simulink model "openloop_simulator"  (R2017a)
settings: Solver=ode4  StartTime=0.0  StopTime=inf  FixedStep=0.1  RelTol=1e-3
libraries: realtime_pacer_lib x1
settings Model: SnapshotBufferSize=1000  SnapshotInterval=1000  Creator=Roshan  LastModifiedBy=rosha
settings RTWCC: SystemTargetFile=sldrt.tlc  TemplateMakefile=sldrt.tmf  Description=Simulink Desktop Real-Time  RTWCompilerOptimization=on
settings CodeAppCC: MaxIdLength=95
settings SimulinkDesktopRealTimeCC: TargetPreCompLibLocation=C:\Program Files\MATLAB\R2017a\toolbox\sldrt\lib\win64  SupportVariableSizeSignals=off

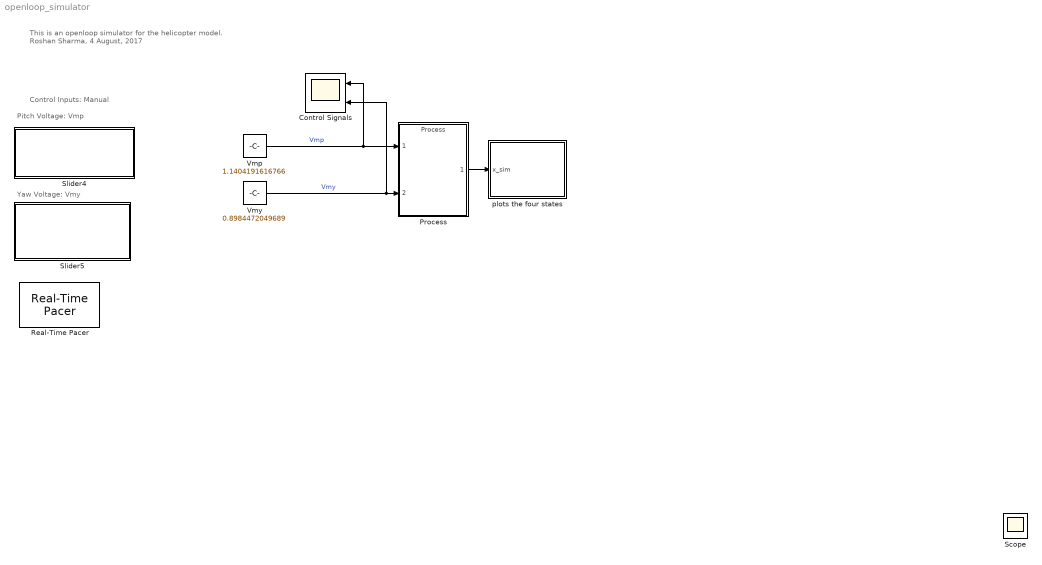
== system openloop_simulator ==
  note: Control Inputs: Manual
  note: This is an openloop simulator
      | for the helicopter model.
      | Roshan Sharma, 4 August, 2017
  note: Pitch Voltage: Vmp
  note: Yaw Voltage: Vmy
  Control Signals : Scope  NumInputPorts=2
  Process : ModelReference  ModelNameDialog=Process  ModelReferenceVersion=1.989  CopyOfModelProtected=on
  Real-Time Pacer : realtime_pacer_lib/Real-Time Pacer  simTimePerRealTime=1
  Slider4 : Subsystem  DialogController=hmiCreateDDGDialog  IsWebBlock=on  mask(MWDashboardBlock){webBlockId=d7fa2b72-57f0-4581-a642-3c1b7216c1b6, webBlockType=slider, ShowInLibBrowser=on, ShowInitialText=on, HMISrcModelName=protected_simulator}
      mask prompts: webBlockId "WebBlock Id"; webBlockType "WebBlock Type"; HMISrcModelName "Source Model"
      mask help: SimulinkHMI:dialogs:SliderDialogDesc
      mask Help: helpview([docroot '/mapfiles/simulink.map'], 'hmi_slider')
      mask Display:
      | if strcmp(get_param(bdroot(gcb),'BlockDiagramType'), 'library')
      |     image([(matlabroot) '/toolbox/simulink/hmi/icons/Slider.png']);
      | end
  Slider5 : Subsystem  DialogController=hmiCreateDDGDialog  IsWebBlock=on  mask(MWDashboardBlock){webBlockId=2da1ea5c-a5f5-4938-b925-ee22b86d0a23, webBlockType=slider, ShowInLibBrowser=on, ShowInitialText=on, HMISrcModelName=protected_simulator}
      mask prompts: webBlockId "WebBlock Id"; webBlockType "WebBlock Type"; HMISrcModelName "Source Model"
      mask help: SimulinkHMI:dialogs:SliderDialogDesc
      mask Help: helpview([docroot '/mapfiles/simulink.map'], 'hmi_slider')
      mask Display:
      | if strcmp(get_param(bdroot(gcb),'BlockDiagramType'), 'library')
      |     image([(matlabroot) '/toolbox/simulink/hmi/icons/Slider.png']);
      | end
  Vmp : Constant  Value=1.1404191616766
  Vmy : Constant  Value=0.8984472049689
  plots the four states : Subsystem
  Scope : Scope
  wires:
  Vmp/1 -> Process/1, Control Signals/1  "Vmp"
  Vmy/1 -> Process/2, Control Signals/2  "Vmy"
  Process/1 -> plots the four states/1(x_sim)

== system openloop_simulator/Slider4 ==

== system openloop_simulator/Slider5 ==

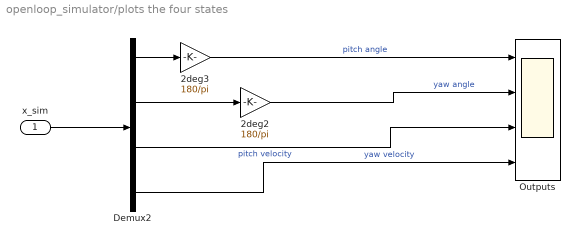
== system openloop_simulator/plots the four states ==
  x_sim : Inport
  2deg2 : Gain  Gain=180/pi
  2deg3 : Gain  Gain=180/pi
  Demux2 : Demux
  Outputs : Scope  NumInputPorts=4
  wires:
  x_sim/1 -> Demux2/1
  Demux2/1 -> 2deg3/1
  Demux2/2 -> 2deg2/1
  2deg3/1 -> Outputs/1  "pitch angle"
  2deg2/1 -> Outputs/2  "yaw angle"
  Demux2/3 -> Outputs/3  "pitch velocity"
  Demux2/4 -> Outputs/4  "yaw velocity"
